simulink model "sin_osc_ver1"  (R2020a)
settings: Solver=ode14x  StartTime=0.0  StopTime=15  FixedStep=0.001  RelTol=1e-3
InitFcn:
  | init_param
StopFcn:
  | plot_out
values from neighbouring files (symbols this model uses):
  deltaT = 2*pi/(n*w)    (= 0.03125)    [init_param.m]
  k = 20    [init_param.m]
  r = 15 * 2*pi/360    (= 0.261799387799)    [init_param.m]
  sb = 1    [init_param.m]
  sf = 0    [init_param.m]
  t_sample = 0.001    [init_param.m]
  td = 0.01    [init_param.m]
  ts = deltaT    (= 0.03125)    [init_param.m]
  u0 = 0    [init_param.m]
  v0 = 0    [init_param.m]
  w = 4*pi    (= 12.5663706144)    [init_param.m]
libraries: dspsrcs4 x52
(part 2 of 2)

== system sin_osc_ver1/head-CPG1 ==
  u_i+1 : Inport
  v_i+1 : Inport  Port=2
  Add : Sum  Inputs=++++
  Add1 : Sum  Inputs=++++
  Constant : Constant  Value=k
  Constant1 : Constant  Value=k
  Constant2 : Constant  Value=r
  Constant3 : Constant  Value=r
  Constant4 : Constant  Value=0
  Discrete Impulse : dspsrcs4/Discrete  Impulse  Delay=round(deltaT/t_sample)+1  SampleTime=t_sample  FrameSample=1  OutputFrames=off  dataType=double  isSigned=on  wordLen=16  udDataType=sfix(16)  fracBitsMode=Best precision  numFracBits=15  OutDataTypeStr=double  LastOutDataTypeStr=double
  Discrete Impulse1 : dspsrcs4/Discrete  Impulse  Delay=round(deltaT/t_sample)  SampleTime=t_sample  FrameSample=1  OutputFrames=off  dataType=double  isSigned=on  wordLen=16  udDataType=sfix(16)  fracBitsMode=Best precision  numFracBits=15  OutDataTypeStr=double  LastOutDataTypeStr=double
  Discrete Impulse2 : dspsrcs4/Discrete  Impulse  Delay=round(deltaT/t_sample)+1  SampleTime=t_sample  FrameSample=1  OutputFrames=off  dataType=double  isSigned=on  wordLen=16  udDataType=sfix(16)  fracBitsMode=Best precision  numFracBits=15  OutDataTypeStr=double  LastOutDataTypeStr=double
  Discrete Impulse3 : dspsrcs4/Discrete  Impulse  Delay=round(deltaT/t_sample)  SampleTime=t_sample  FrameSample=1  OutputFrames=off  dataType=double  isSigned=on  wordLen=16  udDataType=sfix(16)  fracBitsMode=Best precision  numFracBits=15  OutDataTypeStr=double  LastOutDataTypeStr=double
  Gain : Gain  Gain=sb
  Gain1 : Gain  Gain=sf
  Gain2 : Gain  Gain=sf
  Gain3 : Gain  Gain=sb
  Integrator : Integrator  InitialCondition=u0
  Integrator1 : Integrator  InitialCondition=v0
  MATLAB Function : MATLAB Function  TreatAsAtomicUnit=on
  MATLAB Function1 : MATLAB Function  TreatAsAtomicUnit=on
  Product{,1..3} (4 alike) : Product
  Scope : Scope
  Sum : Sum  Inputs=|+-
  Sum1 : Sum  Inputs=|+-
  qu : Subsystem
  w1 : Gain  Gain=w
  w2 : Gain  Gain=-w
  u_i : Outport
  v_i : Outport  Port=2
  wires:
  Constant2/1 -> MATLAB Function/3(r)
  Constant3/1 -> MATLAB Function1/1(r)
  Integrator1/1 -> v_i/1, Sum1/2, MATLAB Function1/3(x), w1/1
  Gain/1 -> Product/1
  Add/1 -> Integrator/1
  w1/1 -> Add/4
  Constant4/1 -> Product1/2
  Constant1/1 -> MATLAB Function1/2(k)
  Product/1 -> Add/2
  qu/1(Out1) -> Product/2
  MATLAB Function/1(y) -> Add/1
  Add1/1 -> Integrator1/1
  Product1/1 -> Add1/3, Scope/1
  Constant/1 -> MATLAB Function/2(k)
  Discrete Impulse1/1 -> Gain1/1
  Gain1/1 -> Product1/1
  w2/1 -> Add1/1
  Discrete Impulse/1 -> Gain/1
  MATLAB Function1/1(y) -> Add1/4
  Discrete Impulse2/1 -> Gain2/1
  Sum/1 -> Product2/2
  Gain2/1 -> Product2/1
  u_i+1/1 -> Sum/1
  Integrator/1 -> u_i/1, Sum/2, MATLAB Function/1(x), w2/1
  Product2/1 -> Add/3
  Discrete Impulse3/1 -> Gain3/1
  Gain3/1 -> Product3/1
  Sum1/1 -> Product3/2
  v_i+1/1 -> Sum1/1
  Product3/1 -> Add1/2

== system sin_osc_ver1/head-CPG1/qu ==
  Step : Step  Time=ts  SampleTime=t_sample
  Step1 : Step  Time=ts + td  SampleTime=t_sample
  Sum : Sum  Inputs=|+-
  Out1 : Outport
  wires:
  Step1/1 -> Sum/2
  Step/1 -> Sum/1
  Sum/1 -> Out1/1

== matlab function sin_osc_ver1/body-CPG6/MATLAB Function1 ==
  data: r input; k input; x input; y output
function y = fcn(r,k,x)
    y = k*(-x/r + (4/pi)*atan(x/r));
% y=0;

== matlab function sin_osc_ver1/body-CPG7/MATLAB Function ==
  data: x input; y output; k input; r input
function y = fcn(x,k,r)
    y = k*(-x/r + (4/pi)*atan(x/r));
% y=0;

== matlab function sin_osc_ver1/body-CPG7/MATLAB Function1 ==
  data: r input; k input; x input; y output
function y = fcn(r,k,x)
    y = k*(-x/r + (4/pi)*atan(x/r));
% y=0;

== matlab function sin_osc_ver1/body-CPG8/MATLAB Function ==
  data: x input; y output; k input; r input
function y = fcn(x,k,r)
    y = k*(-x/r + (4/pi)*atan(x/r));
% y=0;

== matlab function sin_osc_ver1/body-CPG8/MATLAB Function1 ==
  data: r input; k input; x input; y output
function y = fcn(r,k,x)
    y = k*(-x/r + (4/pi)*atan(x/r));
% y=0;

== matlab function sin_osc_ver1/body-CPG9/MATLAB Function ==
  data: x input; y output; k input; r input
function y = fcn(x,k,r)
    y = k*(-x/r + (4/pi)*atan(x/r));
% y=0;

== matlab function sin_osc_ver1/body-CPG9/MATLAB Function1 ==
  data: r input; k input; x input; y output
function y = fcn(r,k,x)
    y = k*(-x/r + (4/pi)*atan(x/r));
% y=0;

== matlab function sin_osc_ver1/body-CPG10/MATLAB Function ==
  data: x input; y output; k input; r input
function y = fcn(x,k,r)
    y = k*(-x/r + (4/pi)*atan(x/r));
% y=0;

== matlab function sin_osc_ver1/head-CPG1/MATLAB Function ==
  data: x input; y output; k input; r input
function y = fcn(x,k,r)
    y = k*(-x/r + (4/pi)*atan(x/r));
% y=0;

== matlab function sin_osc_ver1/body-CPG10/MATLAB Function1 ==
  data: r input; k input; x input; y output
function y = fcn(r,k,x)
    y = k*(-x/r + (4/pi)*atan(x/r));
% y=0;

== matlab function sin_osc_ver1/body-CPG11/MATLAB Function ==
  data: x input; y output; k input; r input
function y = fcn(x,k,r)
    y = k*(-x/r + (4/pi)*atan(x/r));
% y=0;

== matlab function sin_osc_ver1/body-CPG11/MATLAB Function1 ==
  data: r input; k input; x input; y output
function y = fcn(r,k,x)
    y = k*(-x/r + (4/pi)*atan(x/r));
% y=0;

== matlab function sin_osc_ver1/body-CPG12/MATLAB Function ==
  data: x input; y output; k input; r input
function y = fcn(x,k,r)
    y = k*(-x/r + (4/pi)*atan(x/r));
% y=0;

== matlab function sin_osc_ver1/body-CPG12/MATLAB Function1 ==
  data: r input; k input; x input; y output
function y = fcn(r,k,x)
    y = k*(-x/r + (4/pi)*atan(x/r));
% y=0;

== matlab function sin_osc_ver1/body-CPG13/MATLAB Function ==
  data: x input; y output; k input; r input
function y = fcn(x,k,r)
    y = k*(-x/r + (4/pi)*atan(x/r));
% y=0;

== matlab function sin_osc_ver1/body-CPG13/MATLAB Function1 ==
  data: r input; k input; x input; y output
function y = fcn(r,k,x)
    y = k*(-x/r + (4/pi)*atan(x/r));
% y=0;

== matlab function sin_osc_ver1/body-CPG2/MATLAB Function ==
  data: x input; y output; k input; r input
function y = fcn(x,k,r)
    y = k*(-x/r + (4/pi)*atan(x/r));
% y=0;

== matlab function sin_osc_ver1/body-CPG2/MATLAB Function1 ==
  data: r input; k input; x input; y output
function y = fcn(r,k,x)
    y = k*(-x/r + (4/pi)*atan(x/r));
% y=0;

== matlab function sin_osc_ver1/body-CPG3/MATLAB Function ==
  data: x input; y output; k input; r input
function y = fcn(x,k,r)
    y = k*(-x/r + (4/pi)*atan(x/r));
% y=0;

== matlab function sin_osc_ver1/body-CPG3/MATLAB Function1 ==
  data: r input; k input; x input; y output
function y = fcn(r,k,x)
    y = k*(-x/r + (4/pi)*atan(x/r));
% y=0;

== matlab function sin_osc_ver1/body-CPG4/MATLAB Function ==
  data: x input; y output; k input; r input
function y = fcn(x,k,r)
    y = k*(-x/r + (4/pi)*atan(x/r));
% y=0;

== matlab function sin_osc_ver1/body-CPG4/MATLAB Function1 ==
  data: r input; k input; x input; y output
function y = fcn(r,k,x)
    y = k*(-x/r + (4/pi)*atan(x/r));
% y=0;

== matlab function sin_osc_ver1/body-CPG5/MATLAB Function ==
  data: x input; y output; k input; r input
function y = fcn(x,k,r)
    y = k*(-x/r + (4/pi)*atan(x/r));
% y=0;

== matlab function sin_osc_ver1/head-CPG1/MATLAB Function1 ==
  data: r input; k input; x input; y output
function y = fcn(r,k,x)
    y = k*(-x/r + (4/pi)*atan(x/r));
% y=0;

== matlab function sin_osc_ver1/body-CPG5/MATLAB Function1 ==
  data: r input; k input; x input; y output
function y = fcn(r,k,x)
    y = k*(-x/r + (4/pi)*atan(x/r));
% y=0;

== matlab function sin_osc_ver1/body-CPG6/MATLAB Function ==
  data: x input; y output; k input; r input
function y = fcn(x,k,r)
    y = k*(-x/r + (4/pi)*atan(x/r));
% y=0;
